simulink model "hardware_visualization"  (Simulink 7.7)
settings: Solver=FixedStepDiscrete  StartTime=0.0  StopTime=inf  RelTol=1e-3
values from neighbouring files (symbols this model uses):
  Fs = sampRate    [correlation_freq.m]    (also in correlation_freq_w_decimation.m = 8000; fourklpf.m = 8000; plotTandF.m = 1/Ts; step_through_spectrum.m = 48000)
undefined symbols (not defined in the file or in its folder): jet
libraries: dspsnks4 x3, dspsrcs4 x1, dspspect3 x1, dspmtrx3 x1, dspmathops x1
settings Model: Creator=staticd  LastModifiedBy=staticd
settings DebuggingCC: StrictBusMsg=Warning

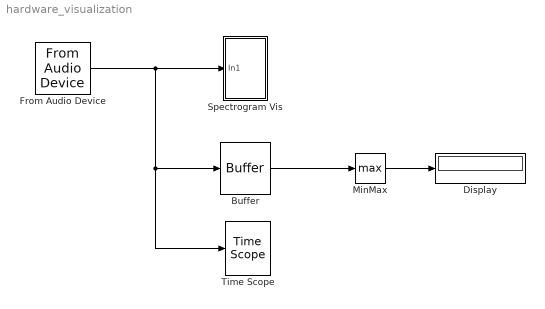
== system hardware_visualization ==
  Buffer : Buffer  N=20480  TreatMby1Signals=One channel
  Display : Display
  From Audio Device : dspsrcs4/From Audio Device  deviceName=Default  numChannels=1  sampleRate=44100  deviceDatatype=Determine from output data type  autoBufferSize=on  bufferSize=4096  queueDuration=1.0  frameSize=1024  outputDatatype=double
  MinMax : MinMax  Function=max
  Spectrogram Vis : Subsystem
  Time Scope : dspsnks4/Time Scope
  wires:
  From Audio Device/1 -> Spectrogram Vis/1(In1), Buffer/1, Time Scope/1
  Buffer/1 -> MinMax/1
  MinMax/1 -> Display/1

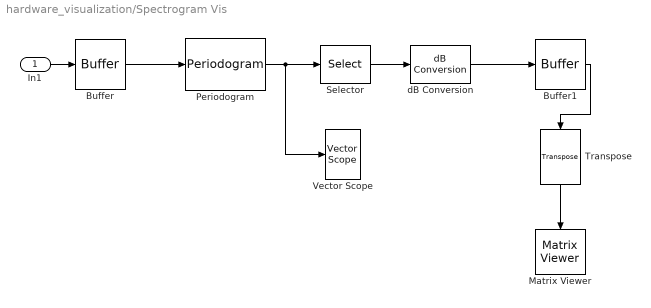
== system hardware_visualization/Spectrogram Vis ==
  In1 : Inport
  Buffer : Buffer  N=256
  Buffer1 : Buffer  V=60  ic=-1
  Matrix Viewer : dspsnks4/Matrix Viewer  ImageParams=off  CMapStr=jet(256)  AxisColorbar=on  AxisParams=off  AxisOrigin=Lower left corner  XLabel=Time Index  YLabel=Frequency Index  ZLabel=dB Magnitude  FigPos=[468 340 380 320]  AxisZoom=off
      settings: YMin=-60  YMax=10
  Periodogram : dspspect3/Periodogram  SystemSampleTime=-1  measurement=Power spectral density  wintype=Hamming  Rs=50  beta=5  winsamp=Periodic  inheritFFT=on  fftsize=256  navg=1  inheritTs=on  Ts=1
  Selector : Selector  InputPortWidth=256  IndexOptions=Index vector (dialog)  Indices=[1:128]  OutputSizes=1
  Transpose : dspmtrx3/Transpose  SystemSampleTime=-1  Hermitian=off  overflowFlag=off
  Vector Scope : dspsnks4/Vector Scope  ScopeProperties=on  Domain=Frequency  HorizSpan=1  DisplayProperties=off  AxisGrid=on  Memory=off  FrameNumber=on  AxisLegend=off  AxisZoom=off  OpenScopeAtSimStart=on  OpenScopeImmediately=off  FigPos=[80 390 380 320]  AxisProperties=off  XUnits=Hertz  XRange=[-Fs/2...Fs/2]  InheritXIncr=on  XIncr=1  XLabel=Time  XLimit=Auto  XMin=0  XMax=1  XStart=0  YUnits=dB  YLabel=Magnitude, dB  LineProperties=off  XAxisParamsVer=6.9
      settings: YMin=-60  YMax=10
  dB Conversion : dspmathops/dB Conversion  SystemSampleTime=-1  dBtype=dB  intype=Power  R=1  fuzz=on
  wires:
  Buffer/1 -> Periodogram/1
  Periodogram/1 -> Selector/1, Vector Scope/1
  Selector/1 -> dB Conversion/1
  dB Conversion/1 -> Buffer1/1
  Buffer1/1 -> Transpose/1
  Transpose/1 -> Matrix Viewer/1
  In1/1 -> Buffer/1
